simulink model "model"  (R2018a)
settings: Solver=VariableStepAuto  StartTime=0.0  StopTime=120  FixedStep=0.01  MaxStep=.001  RelTol=1e-3
libraries: instrumentlib x16, simulink x3
settings Model: Creator=U500304  LastModifiedBy=U500304
settings SolverCC: ZeroCrossAlgorithm=Adaptive
settings DebuggingCC: MaxConsecutiveZCsMsg=warning

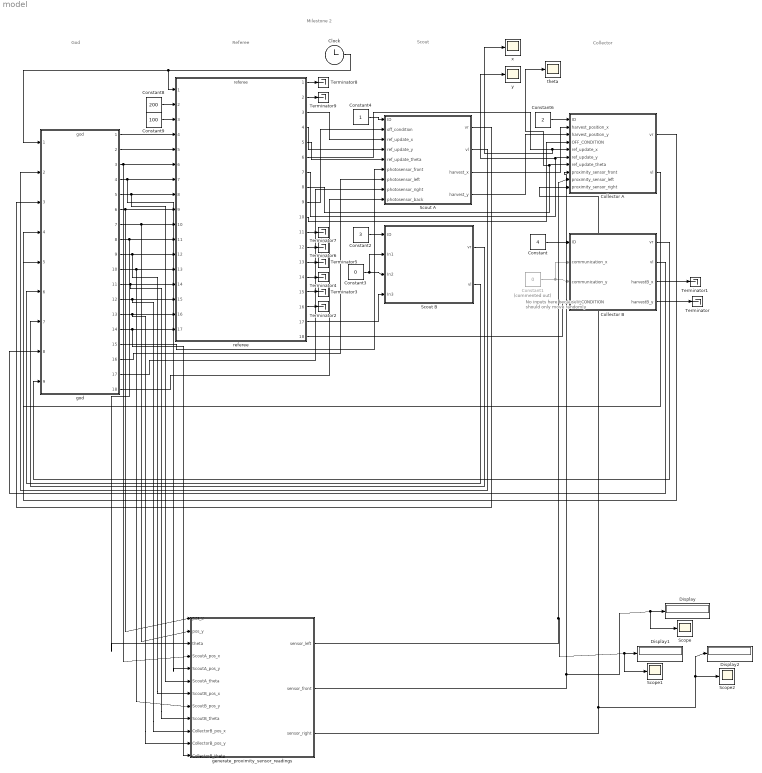
== system model ==
  note: No inputs here because
      | it should only move
      | randomly
  note: Milestone 2
  note: God
  note: Referee
  note: Scout
  note: Collector
  Clock : Clock
  Collector A : Subsystem
  Collector B : Subsystem
  Constant : Constant  Value=4
  Constant1 : Constant  Commented=on  Value=0
  Constant2 : Constant  Value=3
  Constant3 : Constant  Value=0
  Constant4 : Constant
  Constant6 : Constant  Value=2
  Constant8 : Constant  Value=200
  Constant9 : Constant  Value=100
  Display : Display
  Display1 : Display
  Display2 : Display
  Scope : Scope
  Scope1 : Scope
  Scope2 : Scope
  Scout A : Subsystem
  Scout B : Subsystem
  Terminator{,1..9} (10 alike) : Terminator
  generate_proximity_sensor_readings : Subsystem
  god : ModelReference  ModelNameDialog=god  SimulationMode=Normal  ModelReferenceVersion=1.469
  referee : ModelReference  ModelNameDialog=referee  SimulationMode=Normal  ModelReferenceVersion=1.290
  theta : Scope
  x : Scope
  y : Scope
  wires:
  Clock/1 -> god/1, referee/1
  Constant/1 -> Collector B/1(ID)
  Constant1/1 -> Collector B/2(communication_x), Collector B/3(communication_y)
  Constant2/1 -> Scout B/1(ID)
  Constant3/1 -> Scout B/2(In1), Scout B/3(In2)
  Constant4/1 -> Scout A/1(ID)
  Constant6/1 -> Collector A/1(ID)
  Constant8/1 -> referee/2
  Constant9/1 -> referee/3
  god/1 -> referee/4
  god/2 -> referee/5
  god/3 -> generate_proximity_sensor_readings/4(ScoutA_pos_x), referee/6
  god/5 -> generate_proximity_sensor_readings/6(ScoutA_theta), referee/8
  god/6 -> generate_proximity_sensor_readings/1(pos_x), referee/9
  god/7 -> generate_proximity_sensor_readings/2(pos_y), referee/10
  god/8 -> generate_proximity_sensor_readings/3(theta), referee/11
  god/9 -> generate_proximity_sensor_readings/7(ScoutB_pos_x), referee/12
  god/10 -> generate_proximity_sensor_readings/8(ScoutB_pos_y), referee/13
  god/11 -> generate_proximity_sensor_readings/9(ScoutB_theta), referee/14
  god/12 -> generate_proximity_sensor_readings/10(CollectorB_pos_x), referee/15
  god/14 -> generate_proximity_sensor_readings/12(CollectorB_theta), referee/17
  Scout B/2(vl) -> god/6
  Scout B/1(vr) -> god/7
  Collector A/2(vl) -> god/4
  Collector A/1(vr) -> god/5
  Collector B/1(vr) -> god/9
  Collector B/2(vl) -> god/8
  god/13 -> generate_proximity_sensor_readings/11(CollectorB_pos_y), referee/16
  god/4 -> generate_proximity_sensor_readings/5(ScoutA_pos_y), referee/7
  Scout A/1(vr) -> god/3
  Scout A/2(vl) -> god/2
  god/18 -> Scout A/9(photosensor_back)
  god/17 -> Scout A/8(photosensor_right)
  god/16 -> Scout A/7(photosensor_left)
  god/15 -> Scout A/6(photosensor_front)
  Scout A/3(harvest_x) -> Collector A/2(harvest_position_x)
  Scout A/4(harvest_y) -> Collector A/3(harvest_position_y)
  referee/3 -> Scout A/3(ref_update_x)
  referee/4 -> Scout A/4(ref_update_y)
  referee/5 -> Scout A/5(ref_update_theta)
  referee/6 -> x/1, Collector A/5(ref_update_x)
  referee/7 -> y/1, Collector A/6(ref_update_y)
  referee/8 -> theta/1, Collector A/7(ref_update_theta)
  referee/9 -> Scout A/2(off_condition)
  referee/10 -> Collector A/4(OFF_CONDITION)
  referee/18 -> Collector B/4(OFF_CONDITION)
  referee/17 -> Scout B/4(In3)
  generate_proximity_sensor_readings/1(sensor_left) -> Scope1/1, Display1/1, Collector A/9(proximity_sensor_left)
  generate_proximity_sensor_readings/2(sensor_front) -> Scope/1, Display/1, Collector A/8(proximity_sensor_front)
  generate_proximity_sensor_readings/3("sensor_right ") -> Scope2/1, Display2/1, Collector A/10(proximity_sensor_right)
  Collector B/4(harvestB_y) -> Terminator/1
  Collector B/3(harvestB_x) -> Terminator1/1
  referee/16 -> Terminator2/1
  referee/15 -> Terminator3/1
  referee/14 -> Terminator4/1
  referee/13 -> Terminator5/1
  referee/12 -> Terminator6/1
  referee/11 -> Terminator7/1
  referee/2 -> Terminator9/1
  referee/1 -> Terminator8/1

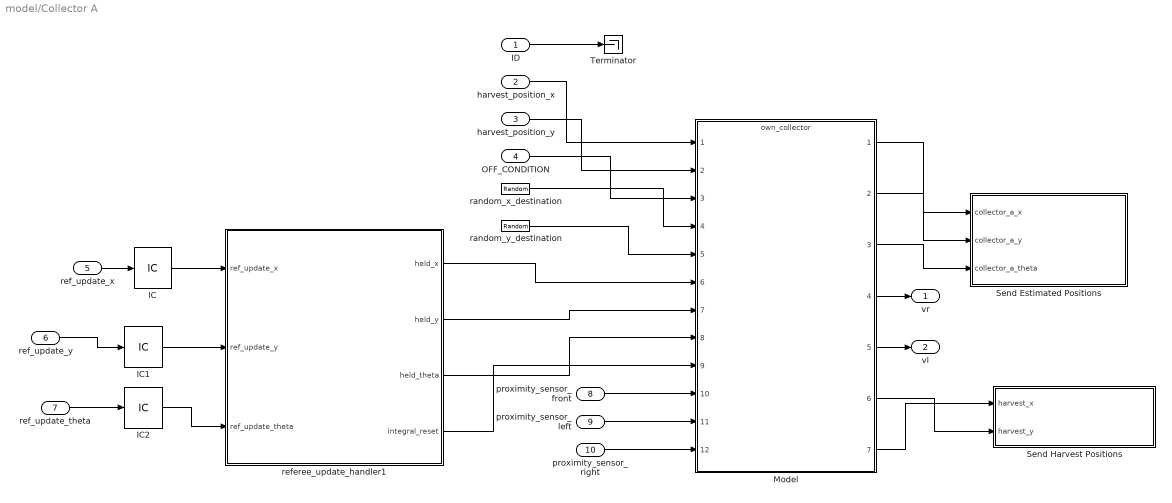
== system model/Collector A ==
  ID : Inport
  harvest_position_x : Inport  Port=2
  harvest_position_y : Inport  Port=3
  OFF_CONDITION : Inport  Port=4  OutDataTypeStr=boolean
  ref_update_x : Inport  Port=5
  ref_update_y : Inport  Port=6
  ref_update_theta : Inport  Port=7
  proximity_sensor_front : Inport  Port=8
  proximity_sensor_left : Inport  Port=9
  proximity_sensor_right : Inport  Port=10
  IC : InitialCondition  Value=0
  IC1 : InitialCondition  Value=49
  IC2 : InitialCondition  Value=0
  Model : ModelReference  ModelNameDialog=own_collector.slx  SimulationMode=Normal  ModelReferenceVersion=1.434
  Send Estimated Positions : Subsystem
  Send Harvest Positions : Subsystem
  Terminator : Terminator
  random_x_destination : UniformRandomNumber  Minimum=-3  Maximum=3  Seed=13  SampleTime=1
  random_y_destination : UniformRandomNumber  Minimum=-3  Maximum=3  Seed=15  SampleTime=1
  referee_update_handler1 : Subsystem
  vr : Outport
  vl : Outport  Port=2
  wires:
  ID/1 -> Terminator/1
  harvest_position_x/1 -> Model/1
  harvest_position_y/1 -> Model/2
  OFF_CONDITION/1 -> Model/3
  random_x_destination/1 -> Model/4
  random_y_destination/1 -> Model/5
  Model/4 -> vr/1
  Model/5 -> vl/1
  Model/1 -> Send Estimated Positions/1(collector_a_x)
  Model/2 -> Send Estimated Positions/2(collector_a_y)
  Model/3 -> Send Estimated Positions/3(collector_a_theta)
  Model/6 -> Send Harvest Positions/2(harvest_y)
  Model/7 -> Send Harvest Positions/1(harvest_x)
  ref_update_x/1 -> IC/1
  ref_update_y/1 -> IC1/1
  ref_update_theta/1 -> IC2/1
  referee_update_handler1/1(held_x) -> Model/6
  referee_update_handler1/2(held_y) -> Model/7
  referee_update_handler1/3(held_theta) -> Model/8
  referee_update_handler1/4(integral_reset) -> Model/9
  IC/1 -> referee_update_handler1/1(ref_update_x)
  IC1/1 -> referee_update_handler1/2(ref_update_y)
  IC2/1 -> referee_update_handler1/3(ref_update_theta)
  proximity_sensor_front/1 -> Model/10
  proximity_sensor_left/1 -> Model/11
  proximity_sensor_right/1 -> Model/12

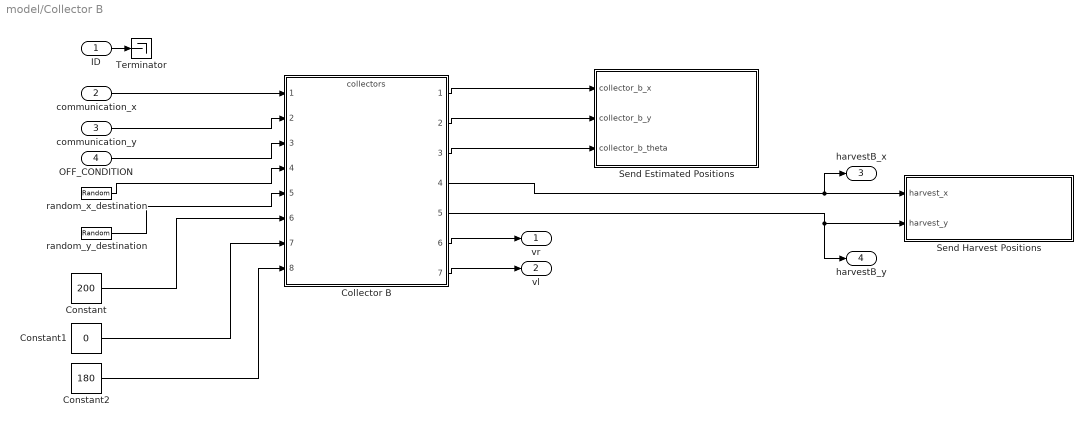
== system model/Collector B ==
  ID : Inport
  communication_x : Inport  Port=2
  communication_y : Inport  Port=3
  OFF_CONDITION : Inport  Port=4  OutDataTypeStr=boolean
  Collector B : ModelReference  ModelNameDialog=collectors  SimulationMode=Normal  ModelReferenceVersion=1.299
  Constant : Constant  Value=200
  Constant1 : Constant  Value=0
  Constant2 : Constant  Value=180
  Send Estimated Positions : Subsystem
  Send Harvest Positions : Subsystem
  Terminator : Terminator
  random_x_destination : UniformRandomNumber  Minimum=0  Maximum=199  Seed=18  SampleTime=1
  random_y_destination : UniformRandomNumber  Minimum=0  Maximum=99  Seed=19  SampleTime=1
  vr : Outport
  vl : Outport  Port=2
  harvestB_x : Outport  Port=3
  harvestB_y : Outport  Port=4
  wires:
  Collector B/2 -> Send Estimated Positions/2(collector_b_y)
  communication_x/1 -> Collector B/1
  Collector B/3 -> Send Estimated Positions/3(collector_b_theta)
  random_y_destination/1 -> Collector B/5
  random_x_destination/1 -> Collector B/4
  Collector B/1 -> Send Estimated Positions/1(collector_b_x)
  OFF_CONDITION/1 -> Collector B/3
  communication_y/1 -> Collector B/2
  ID/1 -> Terminator/1
  Collector B/6 -> vr/1
  Collector B/7 -> vl/1
  Collector B/4 -> harvestB_x/1, Send Harvest Positions/1(harvest_x)
  Collector B/5 -> harvestB_y/1, Send Harvest Positions/2(harvest_y)
  Constant/1 -> Collector B/6
  Constant1/1 -> Collector B/7
  Constant2/1 -> Collector B/8

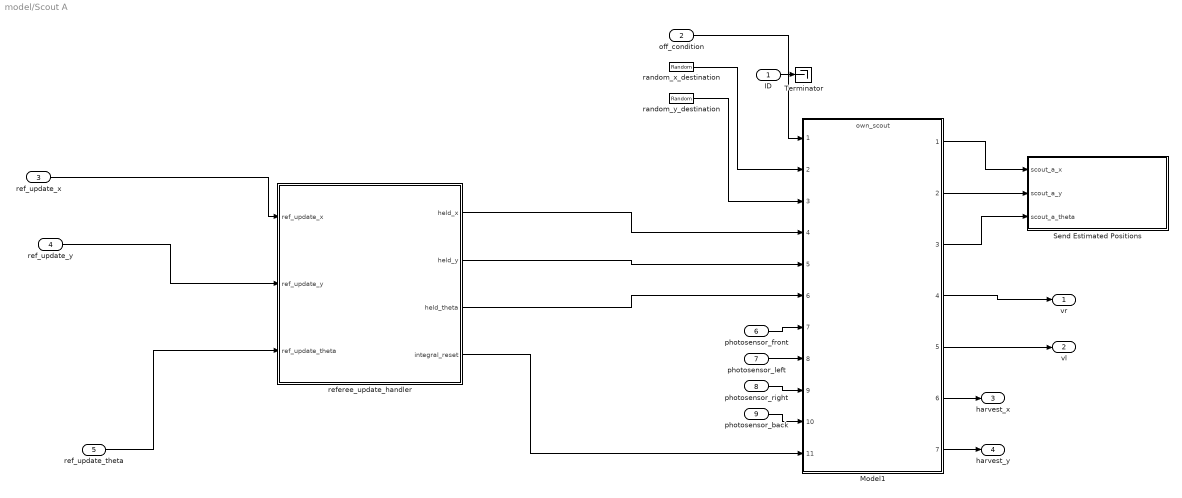
== system model/Scout A ==
  ID : Inport
  off_condition : Inport  Port=2  OutDataTypeStr=boolean
  ref_update_x : Inport  Port=3
  ref_update_y : Inport  Port=4
  ref_update_theta : Inport  Port=5
  photosensor_front : Inport  Port=6
  photosensor_left : Inport  Port=7
  photosensor_right : Inport  Port=8
  photosensor_back : Inport  Port=9
  Model1 : ModelReference  ModelNameDialog=own_scout.slx  SimulationMode=Normal  ModelReferenceVersion=1.295
  Send Estimated Positions : Subsystem
  Terminator : Terminator
  random_x_destination : UniformRandomNumber  Minimum=0  Maximum=199  Seed=11  SampleTime=1
  random_y_destination : UniformRandomNumber  Minimum=0  Maximum=99  Seed=12  SampleTime=1
  referee_update_handler : Subsystem
  vr : Outport
  vl : Outport  Port=2
  harvest_x : Outport  Port=3
  harvest_y : Outport  Port=4
  wires:
  off_condition/1 -> Model1/1
  random_x_destination/1 -> Model1/2
  random_y_destination/1 -> Model1/3
  ID/1 -> Terminator/1
  Model1/1 -> Send Estimated Positions/1(scout_a_x)
  Model1/2 -> Send Estimated Positions/2(scout_a_y)
  Model1/3 -> Send Estimated Positions/3(scout_a_theta)
  Model1/4 -> vr/1
  Model1/5 -> vl/1
  Model1/7 -> harvest_y/1
  Model1/6 -> harvest_x/1
  photosensor_back/1 -> Model1/10
  photosensor_right/1 -> Model1/9
  photosensor_left/1 -> Model1/8
  photosensor_front/1 -> Model1/7
  ref_update_x/1 -> referee_update_handler/1(ref_update_x)
  ref_update_y/1 -> referee_update_handler/2(ref_update_y)
  ref_update_theta/1 -> referee_update_handler/3(ref_update_theta)
  referee_update_handler/1(held_x) -> Model1/4
  referee_update_handler/2(held_y) -> Model1/5
  referee_update_handler/3(held_theta) -> Model1/6
  referee_update_handler/4(integral_reset) -> Model1/11

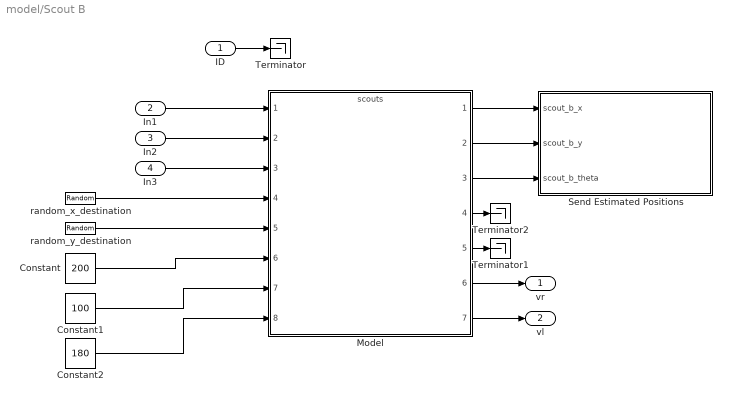
== system model/Scout B ==
  ID : Inport
  In1 : Inport  Port=2
  In2 : Inport  Port=3
  In3 : Inport  Port=4  OutDataTypeStr=boolean
  Constant : Constant  Value=200
  Constant1 : Constant  Value=100
  Constant2 : Constant  Value=180
  Model : ModelReference  ModelNameDialog=scouts.slx  SimulationMode=Normal  ModelReferenceVersion=1.251
  Send Estimated Positions : Subsystem
  Terminator : Terminator
  Terminator1 : Terminator
  Terminator2 : Terminator
  random_x_destination : UniformRandomNumber  Minimum=0  Maximum=199  Seed=16  SampleTime=1
  random_y_destination : UniformRandomNumber  Minimum=0  Maximum=99  Seed=17  SampleTime=1
  vr : Outport
  vl : Outport  Port=2
  wires:
  random_y_destination/1 -> Model/5
  random_x_destination/1 -> Model/4
  In3/1 -> Model/3
  Model/2 -> Send Estimated Positions/2(scout_b_y)
  Model/1 -> Send Estimated Positions/1(scout_b_x)
  In1/1 -> Model/1
  In2/1 -> Model/2
  Model/3 -> Send Estimated Positions/3(scout_b_theta)
  ID/1 -> Terminator/1
  Model/6 -> vr/1
  Model/7 -> vl/1
  Model/4 -> Terminator2/1
  Model/5 -> Terminator1/1
  Constant/1 -> Model/6
  Constant1/1 -> Model/7
  Constant2/1 -> Model/8

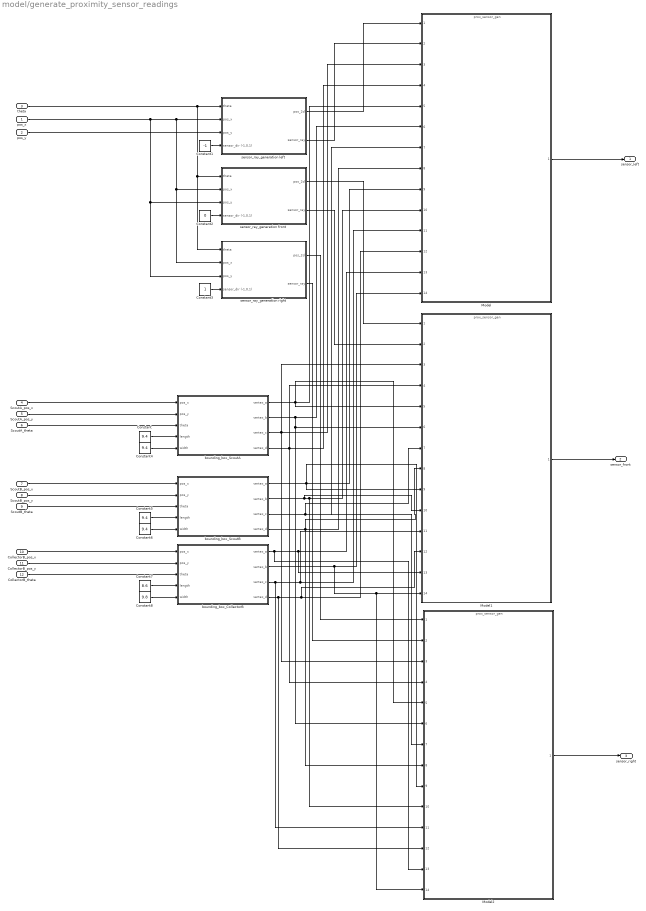
== system model/generate_proximity_sensor_readings ==
  pos_x : Inport
  pos_y : Inport  Port=2
  theta : Inport  Port=3
  ScoutA_pos_x : Inport  Port=4
  ScoutA_pos_y : Inport  Port=5
  ScoutA_theta : Inport  Port=6
  ScoutB_pos_x : Inport  Port=7
  ScoutB_pos_y : Inport  Port=8
  ScoutB_theta : Inport  Port=9
  CollectorB_pos_x : Inport  Port=10
  CollectorB_pos_y : Inport  Port=11
  CollectorB_theta : Inport  Port=12
  Constant{,4..6} (4 alike) : Constant  Value=9.4
  Constant1 : Constant  Value=-1
  Constant2 : Constant  Value=0
  Constant3 : Constant
  Constant7 : Constant  Value=8.6
  Constant8 : Constant  Value=9.8
  Model : ModelReference  ModelNameDialog=prox_sensor_gen  SimulationMode=Normal  ModelReferenceVersion=1.2
  Model1 : ModelReference  ModelNameDialog=prox_sensor_gen  SimulationMode=Normal  ModelReferenceVersion=1.2
  Model2 : ModelReference  ModelNameDialog=prox_sensor_gen  SimulationMode=Normal  ModelReferenceVersion=1.2
  bounding_box_CollectorB : Subsystem
  bounding_box_ScoutA : Subsystem
  bounding_box_ScoutB : Subsystem
  sensor_ray_generation front : Subsystem
  sensor_ray_generation left : Subsystem
  sensor_ray_generation right : Subsystem
  sensor_left : Outport
  sensor_front : Outport  Port=2
  "sensor_right " : Outport  Port=3
  wires:
  theta/1 -> sensor_ray_generation right/1("theta "), sensor_ray_generation front/1("theta "), sensor_ray_generation left/1("theta ")
  bounding_box_CollectorB/2(vertex_b) -> Model/14, Model2/14, Model1/14
  Constant2/1 -> sensor_ray_generation front/4("sensor_dir (-1,0,1) ")
  Model2/1 -> "sensor_right "/1
  bounding_box_ScoutB/4(vertex_d) -> Model2/8, Model1/8, Model/8
  Constant8/1 -> bounding_box_CollectorB/5(width)
  bounding_box_ScoutA/1(vertex_a) -> Model2/5, Model1/5, Model/5
  bounding_box_CollectorB/3(vertex_c) -> Model2/11, Model1/11, Model/11
  ScoutB_theta/1 -> bounding_box_ScoutB/3(theta)
  Constant5/1 -> bounding_box_ScoutB/4(length)
  ScoutA_pos_x/1 -> bounding_box_ScoutA/1(pos_x)
  bounding_box_ScoutA/3(vertex_c) -> Model2/3, Model1/3, Model/3
  Constant6/1 -> bounding_box_ScoutB/5(width)
  Constant1/1 -> sensor_ray_generation left/4("sensor_dir (-1,0,1) ")
  bounding_box_CollectorB/1(vertex_a) -> Model2/13, Model1/13, Model/13
  bounding_box_ScoutA/4(vertex_d) -> Model2/4, Model1/4, Model/4
  sensor_ray_generation front/1(pos_2d) -> Model1/1
  sensor_ray_generation left/2("sensor_ray ") -> Model/2
  bounding_box_CollectorB/4(vertex_d) -> Model2/12, Model1/12, Model/12
  ScoutB_pos_y/1 -> bounding_box_ScoutB/2(pos_y)
  Model/1 -> sensor_left/1
  pos_y/1 -> sensor_ray_generation left/3(pos_y)
  bounding_box_ScoutB/2(vertex_b) -> Model1/10, Model2/10, Model/10
  Model1/1 -> sensor_front/1
  bounding_box_ScoutB/1(vertex_a) -> Model2/9, Model1/9, Model/9
  bounding_box_ScoutA/2(vertex_b) -> Model/6, Model2/6, Model1/6
  bounding_box_ScoutB/3(vertex_c) -> Model2/7, Model1/7, Model/7
  sensor_ray_generation right/2("sensor_ray ") -> Model2/2
  ScoutA_pos_y/1 -> bounding_box_ScoutA/2(pos_y)
  CollectorB_theta/1 -> bounding_box_CollectorB/3(theta)
  pos_x/1 -> sensor_ray_generation right/3(pos_y), sensor_ray_generation front/3(pos_y), sensor_ray_generation right/2(pos_x), sensor_ray_generation front/2(pos_x), sensor_ray_generation left/2(pos_x)
  sensor_ray_generation right/1(pos_2d) -> Model2/1
  Constant4/1 -> bounding_box_ScoutA/5(width)
  CollectorB_pos_x/1 -> bounding_box_CollectorB/1(pos_x)
  Constant/1 -> bounding_box_ScoutA/4(length)
  CollectorB_pos_y/1 -> bounding_box_CollectorB/2(pos_y)
  Constant7/1 -> bounding_box_CollectorB/4(length)
  ScoutA_theta/1 -> bounding_box_ScoutA/3(theta)
  ScoutB_pos_x/1 -> bounding_box_ScoutB/1(pos_x)
  Constant3/1 -> sensor_ray_generation right/4("sensor_dir (-1,0,1) ")
  sensor_ray_generation left/1(pos_2d) -> Model/1
  sensor_ray_generation front/2("sensor_ray ") -> Model1/2

== system model/Collector A/Send Estimated Positions ==
  note: Collector
  collector_a_x : Inport
  collector_a_y : Inport  Port=2
  collector_a_theta : Inport  Port=3
  Rate Transition : RateTransition  OutPortSampleTime=0.05
  Rate Transition1 : RateTransition  OutPortSampleTime=0.05
  Rate Transition2 : RateTransition  OutPortSampleTime=0.05
  tcp_send_collector_a_theta : instrumentlib/TCP//IP Send  Host=localhost  Port=50006  EnableBlockingMode=off  Timeout=1  ByteOrder=LittleEndian  TransferDelay=on
      settings: SourceProductName=Instrument Control Toolbox
  tcp_send_collector_a_x : instrumentlib/TCP//IP Send  Host=localhost  Port=50004  EnableBlockingMode=off  Timeout=1  ByteOrder=LittleEndian  TransferDelay=on
      settings: SourceProductName=Instrument Control Toolbox
  tcp_send_collector_a_y : instrumentlib/TCP//IP Send  Host=localhost  Port=50005  EnableBlockingMode=off  Timeout=1  ByteOrder=LittleEndian  TransferDelay=on
      settings: SourceProductName=Instrument Control Toolbox
  wires:
  collector_a_x/1 -> Rate Transition/1
  collector_a_y/1 -> Rate Transition1/1
  collector_a_theta/1 -> Rate Transition2/1
  Rate Transition/1 -> tcp_send_collector_a_x/1
  Rate Transition1/1 -> tcp_send_collector_a_y/1
  Rate Transition2/1 -> tcp_send_collector_a_theta/1

== system model/Collector A/Send Harvest Positions ==
  note: Collector
  harvest_x : Inport
  harvest_y : Inport  Port=2
  Rate Transition3 : RateTransition  OutPortSampleTime=0.5
  Rate Transition4 : RateTransition  OutPortSampleTime=0.5
  tcp_send_harvest_a_x : instrumentlib/TCP//IP Send  Host=localhost  Port=50025  EnableBlockingMode=off  Timeout=1  ByteOrder=LittleEndian  TransferDelay=on
      settings: SourceProductName=Instrument Control Toolbox
  tcp_send_harvest_a_y : instrumentlib/TCP//IP Send  Host=localhost  Port=50026  EnableBlockingMode=off  Timeout=1  ByteOrder=LittleEndian  TransferDelay=on
      settings: SourceProductName=Instrument Control Toolbox
  wires:
  Rate Transition3/1 -> tcp_send_harvest_a_x/1
  harvest_x/1 -> Rate Transition3/1
  harvest_y/1 -> Rate Transition4/1
  Rate Transition4/1 -> tcp_send_harvest_a_y/1

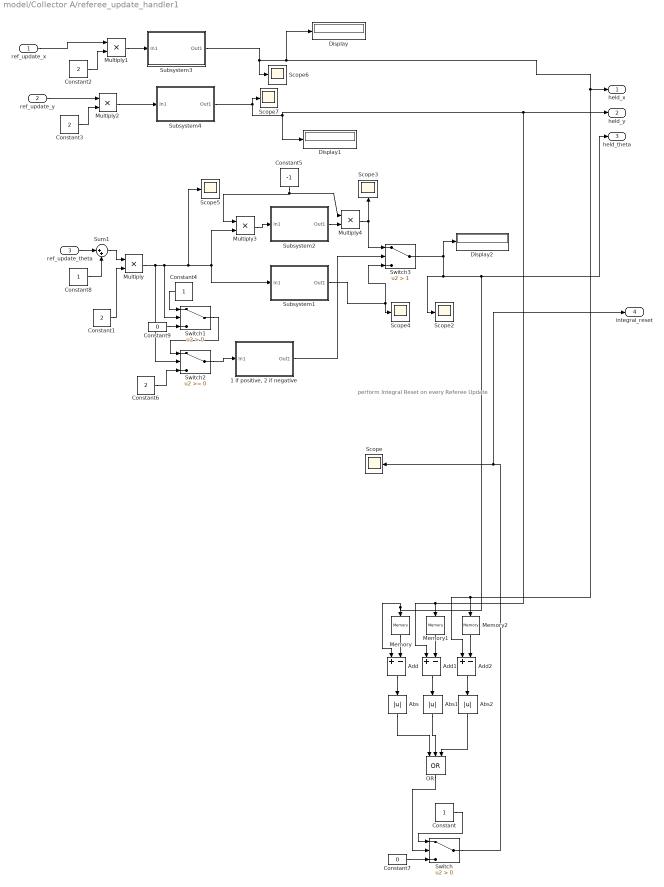
== system model/Collector A/referee_update_handler1 ==
  note: perform
      | Integral
      | Reset on
      | every
      | Referee
      | Update
  ref_update_x : Inport
  ref_update_y : Inport  Port=2
  ref_update_theta : Inport  Port=3
  "1 if positive, 2 if negative" : Subsystem
  Abs : Abs
  Abs1 : Abs
  Abs2 : Abs
  Add : Sum  Inputs=+-
  Add1 : Sum  Inputs=+-
  Add2 : Sum  Inputs=+-
  Constant : Constant
  Constant{1..3,6} (4 alike) : Constant  Value=2
  Constant4 : Constant
  Constant5 : Constant  Value=-1
  Constant7 : Constant  Value=0
  Constant8 : Constant
  Constant9 : Constant  Value=0
  Display : Display
  Display1 : Display
  Display2 : Display
  Memory : Memory
  Memory1 : Memory
  Memory2 : Memory
  Multiply{,1..4} (5 alike) : Product
  OR : Logic  Operator=OR  Inputs=3  IconShape=distinctive  AllPortsSameDT=off  OutDataTypeStr=boolean
  Scope{,2..7} (7 alike) : Scope
  Subsystem1 : Subsystem
  Subsystem2 : Subsystem
  Subsystem3 : Subsystem
  Subsystem4 : Subsystem
  Sum1 : Sum  Inputs=|++
  Switch : Switch  Criteria=u2 > Threshold
  Switch1 : Switch  Criteria=u2 > Threshold
  Switch2 : Switch
  Switch3 : Switch  Criteria=u2 > Threshold  Threshold=1
  held_x : Outport
  held_y : Outport  Port=2
  held_theta : Outport  Port=3
  integral_reset : Outport  Port=4
  wires:
  Multiply1/1 -> Subsystem3/1(In1)
  Add/1 -> Abs/1
  Subsystem3/1(Out1) -> Scope6/1, held_x/1, Add2/1, Memory2/1, Display/1
  Constant1/1 -> Multiply/2
  Subsystem2/1(Out1) -> Multiply4/2
  Multiply3/1 -> Subsystem2/1(In1)
  Multiply/1 -> Switch2/2, Switch1/2, Multiply3/2, Subsystem1/1(In1), Scope5/1
  Subsystem4/1(Out1) -> held_y/1, Add1/1, Memory1/1, Display1/1, Scope7/1
  Constant6/1 -> Switch2/3
  Add2/1 -> Abs2/1
  Memory2/1 -> Add2/2
  Constant3/1 -> Multiply2/2
  Switch3/1 -> Scope2/1, held_theta/1, Add/1, Memory/1, Display2/1
  "1 if positive, 2 if negative"/1(Out1) -> Switch3/2
  Constant2/1 -> Multiply1/2
  Constant5/1 -> Multiply4/1, Multiply3/1
  Switch1/1 -> Switch2/1
  Multiply4/1 -> Scope3/1, Switch3/1
  Sum1/1 -> Multiply/1
  Switch/1 -> integral_reset/1, Scope/1
  Abs2/1 -> OR/3
  Multiply2/1 -> Subsystem4/1(In1)
  Constant/1 -> Switch/1
  Subsystem1/1(Out1) -> Switch3/3, Scope4/1
  Memory/1 -> Add/2
  ref_update_x/1 -> Multiply1/1
  Abs/1 -> OR/1
  ref_update_theta/1 -> Sum1/1
  ref_update_y/1 -> Multiply2/1
  OR/1 -> Switch/2
  Abs1/1 -> OR/2
  Constant8/1 -> Sum1/2
  Add1/1 -> Abs1/1
  Memory1/1 -> Add1/2
  Constant4/1 -> Switch1/1
  Switch2/1 -> "1 if positive, 2 if negative"/1(In1)
  Constant7/1 -> Switch/3
  Constant9/1 -> Switch1/3

== system model/Collector B/Send Estimated Positions ==
  note: Collector
  collector_b_x : Inport
  collector_b_y : Inport  Port=2
  collector_b_theta : Inport  Port=3
  Rate Transition10 : RateTransition  OutPortSampleTime=0.1
  Rate Transition11 : RateTransition  OutPortSampleTime=0.1
  Rate Transition9 : RateTransition  OutPortSampleTime=0.1
  tcp_send_collector_b_theta : instrumentlib/TCP//IP Send  Host=localhost  Port=50012  EnableBlockingMode=off  Timeout=1  ByteOrder=LittleEndian  TransferDelay=on
      settings: SourceProductName=Instrument Control Toolbox
  tcp_send_collector_b_x : instrumentlib/TCP//IP Send  Host=localhost  Port=50010  EnableBlockingMode=off  Timeout=1  ByteOrder=LittleEndian  TransferDelay=on
      settings: SourceProductName=Instrument Control Toolbox
  tcp_send_collector_b_y : instrumentlib/TCP//IP Send  Host=localhost  Port=50011  EnableBlockingMode=off  Timeout=1  ByteOrder=LittleEndian  TransferDelay=on
      settings: SourceProductName=Instrument Control Toolbox
  wires:
  collector_b_x/1 -> Rate Transition9/1
  collector_b_y/1 -> Rate Transition10/1
  collector_b_theta/1 -> Rate Transition11/1
  Rate Transition9/1 -> tcp_send_collector_b_x/1
  Rate Transition10/1 -> tcp_send_collector_b_y/1
  Rate Transition11/1 -> tcp_send_collector_b_theta/1

== system model/Collector B/Send Harvest Positions ==
  note: Collector
  harvest_x : Inport
  harvest_y : Inport  Port=2
  Rate Transition3 : RateTransition  OutPortSampleTime=0.5
  Rate Transition4 : RateTransition  OutPortSampleTime=0.5
  tcp_send_collector_b_theta2 : instrumentlib/TCP//IP Send  Host=localhost  Port=50028  EnableBlockingMode=off  Timeout=1  ByteOrder=LittleEndian  TransferDelay=on
      settings: SourceProductName=Instrument Control Toolbox
  tcp_send_harvest_b_x : instrumentlib/TCP//IP Send  Host=localhost  Port=50027  EnableBlockingMode=off  Timeout=1  ByteOrder=LittleEndian  TransferDelay=on
      settings: SourceProductName=Instrument Control Toolbox
  wires:
  Rate Transition3/1 -> tcp_send_harvest_b_x/1
  harvest_x/1 -> Rate Transition3/1
  harvest_y/1 -> Rate Transition4/1
  Rate Transition4/1 -> tcp_send_collector_b_theta2/1

== system model/Scout A/Send Estimated Positions ==
  note: Scout
  scout_a_x : Inport
  scout_a_y : Inport  Port=2
  scout_a_theta : Inport  Port=3
  Rate Transition5 : RateTransition  OutPortSampleTime=0.05
  Rate Transition6 : RateTransition  OutPortSampleTime=0.05
  Rate Transition7 : RateTransition  OutPortSampleTime=0.05
  tcp_send_scout_a_theta : instrumentlib/TCP//IP Send  Host=localhost  Port=50003  EnableBlockingMode=off  Timeout=1  ByteOrder=LittleEndian  TransferDelay=on
      settings: SourceProductName=Instrument Control Toolbox
  tcp_send_scout_a_x : instrumentlib/TCP//IP Send  Host=localhost  Port=50001  EnableBlockingMode=off  Timeout=1  ByteOrder=LittleEndian  TransferDelay=on
      settings: SourceProductName=Instrument Control Toolbox
  tcp_send_scout_a_y : instrumentlib/TCP//IP Send  Host=localhost  Port=50002  EnableBlockingMode=off  Timeout=1  ByteOrder=LittleEndian  TransferDelay=on
      settings: SourceProductName=Instrument Control Toolbox
  wires:
  scout_a_x/1 -> Rate Transition5/1
  scout_a_y/1 -> Rate Transition6/1
  scout_a_theta/1 -> Rate Transition7/1
  Rate Transition5/1 -> tcp_send_scout_a_x/1
  Rate Transition6/1 -> tcp_send_scout_a_y/1
  Rate Transition7/1 -> tcp_send_scout_a_theta/1

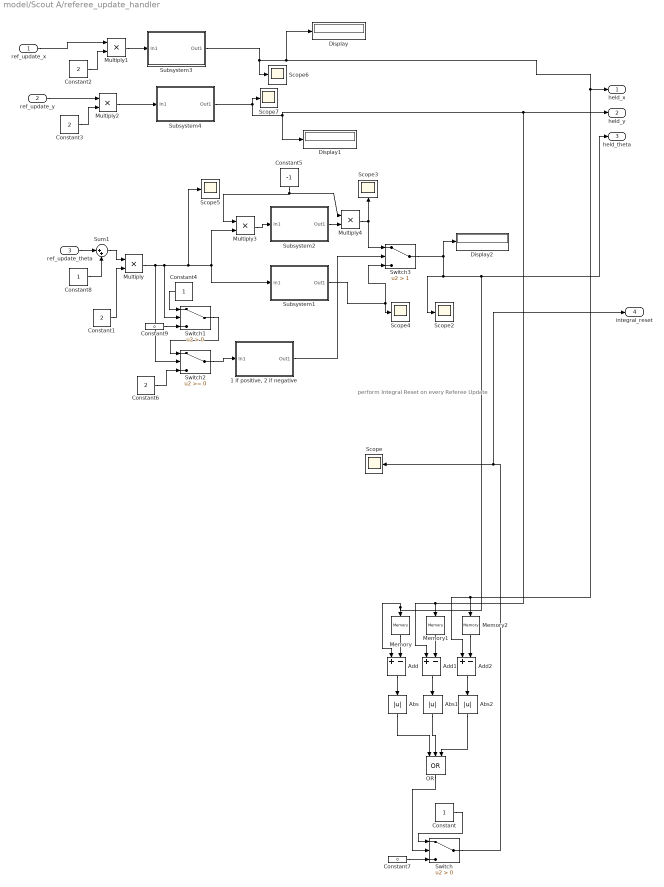
== system model/Scout A/referee_update_handler ==
  note: perform
      | Integral
      | Reset on
      | every
      | Referee
      | Update
  ref_update_x : Inport
  ref_update_y : Inport  Port=2
  ref_update_theta : Inport  Port=3
  "1 if positive, 2 if negative" : Subsystem
  Abs : Abs
  Abs1 : Abs
  Abs2 : Abs
  Add : Sum  Inputs=+-
  Add1 : Sum  Inputs=+-
  Add2 : Sum  Inputs=+-
  Constant : Constant
  Constant{1..3,6} (4 alike) : Constant  Value=2
  Constant4 : Constant
  Constant5 : Constant  Value=-1
  Constant7 : Constant  Value=0
  Constant8 : Constant
  Constant9 : Constant  Value=0
  Display : Display
  Display1 : Display
  Display2 : Display
  Memory : Memory
  Memory1 : Memory
  Memory2 : Memory
  Multiply{,1..4} (5 alike) : Product
  OR : Logic  Operator=OR  Inputs=3  IconShape=distinctive  AllPortsSameDT=off  OutDataTypeStr=boolean
  Scope{,2..7} (7 alike) : Scope
  Subsystem1 : Subsystem
  Subsystem2 : Subsystem
  Subsystem3 : Subsystem
  Subsystem4 : Subsystem
  Sum1 : Sum  Inputs=|++
  Switch : Switch  Criteria=u2 > Threshold
  Switch1 : Switch  Criteria=u2 > Threshold
  Switch2 : Switch
  Switch3 : Switch  Criteria=u2 > Threshold  Threshold=1
  held_x : Outport
  held_y : Outport  Port=2
  held_theta : Outport  Port=3
  integral_reset : Outport  Port=4
  wires:
  Multiply1/1 -> Subsystem3/1(In1)
  Add/1 -> Abs/1
  Subsystem3/1(Out1) -> Scope6/1, held_x/1, Add2/1, Memory2/1, Display/1
  Constant1/1 -> Multiply/2
  Subsystem2/1(Out1) -> Multiply4/2
  Multiply3/1 -> Subsystem2/1(In1)
  Multiply/1 -> Switch2/2, Switch1/2, Multiply3/2, Subsystem1/1(In1), Scope5/1
  Subsystem4/1(Out1) -> held_y/1, Add1/1, Memory1/1, Display1/1, Scope7/1
  Constant6/1 -> Switch2/3
  Add2/1 -> Abs2/1
  Memory2/1 -> Add2/2
  Constant3/1 -> Multiply2/2
  Switch3/1 -> Scope2/1, held_theta/1, Add/1, Memory/1, Display2/1
  "1 if positive, 2 if negative"/1(Out1) -> Switch3/2
  Constant2/1 -> Multiply1/2
  Constant5/1 -> Multiply4/1, Multiply3/1
  Switch1/1 -> Switch2/1
  Multiply4/1 -> Scope3/1, Switch3/1
  Sum1/1 -> Multiply/1
  Switch/1 -> integral_reset/1, Scope/1
  Abs2/1 -> OR/3
  Multiply2/1 -> Subsystem4/1(In1)
  Constant/1 -> Switch/1
  Subsystem1/1(Out1) -> Switch3/3, Scope4/1
  Memory/1 -> Add/2
  ref_update_x/1 -> Multiply1/1
  Abs/1 -> OR/1
  ref_update_theta/1 -> Sum1/1
  ref_update_y/1 -> Multiply2/1
  OR/1 -> Switch/2
  Abs1/1 -> OR/2
  Constant8/1 -> Sum1/2
  Add1/1 -> Abs1/1
  Memory1/1 -> Add1/2
  Constant4/1 -> Switch1/1
  Switch2/1 -> "1 if positive, 2 if negative"/1(In1)
  Constant7/1 -> Switch/3
  Constant9/1 -> Switch1/3

== system model/Scout B/Send Estimated Positions ==
  note: Scout
  scout_b_x : Inport
  scout_b_y : Inport  Port=2
  scout_b_theta : Inport  Port=3
  Rate Transition3 : RateTransition  OutPortSampleTime=0.1
  Rate Transition4 : RateTransition  OutPortSampleTime=0.1
  Rate Transition8 : RateTransition  OutPortSampleTime=0.1
  tcp_send_scout_b_theta : instrumentlib/TCP//IP Send  Host=localhost  Port=50009  EnableBlockingMode=off  Timeout=1  ByteOrder=LittleEndian  TransferDelay=on
      settings: SourceProductName=Instrument Control Toolbox
  tcp_send_scout_b_x : instrumentlib/TCP//IP Send  Host=localhost  Port=50007  EnableBlockingMode=off  Timeout=1  ByteOrder=LittleEndian  TransferDelay=on
      settings: SourceProductName=Instrument Control Toolbox
  tcp_send_scout_b_y : instrumentlib/TCP//IP Send  Host=localhost  Port=50008  EnableBlockingMode=off  Timeout=1  ByteOrder=LittleEndian  TransferDelay=on
      settings: SourceProductName=Instrument Control Toolbox
  wires:
  scout_b_theta/1 -> Rate Transition8/1
  scout_b_y/1 -> Rate Transition4/1
  scout_b_x/1 -> Rate Transition3/1
  Rate Transition3/1 -> tcp_send_scout_b_x/1
  Rate Transition4/1 -> tcp_send_scout_b_y/1
  Rate Transition8/1 -> tcp_send_scout_b_theta/1

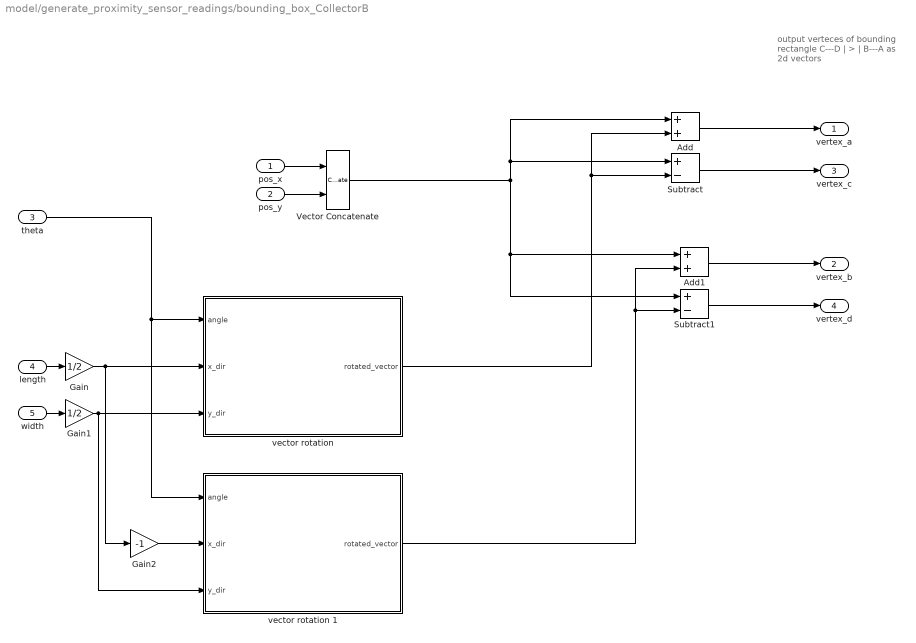
== system model/generate_proximity_sensor_readings/bounding_box_CollectorB ==
  note: output verteces of
      | bounding rectangle
      | C---D
      | |  >  |
      | B---A  as 2d vectors
  pos_x : Inport
  pos_y : Inport  Port=2
  theta : Inport  Port=3
  length : Inport  Port=4
  width : Inport  Port=5
  Add : Sum
  Add1 : Sum
  Gain : Gain  Gain=1/2
  Gain1 : Gain  Gain=1/2
  Gain2 : Gain  Gain=-1
  Subtract : Sum  Inputs=+-
  Subtract1 : Sum  Inputs=+-
  Vector Concatenate : Concatenate
  "vector rotation " : Subsystem
  vector rotation 1 : Subsystem
  vertex_a : Outport
  vertex_b : Outport  Port=2
  vertex_c : Outport  Port=3
  vertex_d : Outport  Port=4
  wires:
  Subtract1/1 -> vertex_d/1
  Add1/1 -> vertex_b/1
  Subtract/1 -> vertex_c/1
  Add/1 -> vertex_a/1
  vector rotation 1/1("rotated_vector ") -> Add1/2, Subtract1/2
  "vector rotation "/1("rotated_vector ") -> Add/2, Subtract/2
  Vector Concatenate/1 -> Add/1, Subtract/1, Add1/1, Subtract1/1
  Gain1/1 -> "vector rotation "/3(y_dir), vector rotation 1/3(y_dir)
  Gain2/1 -> vector rotation 1/2(x_dir)
  Gain/1 -> "vector rotation "/2(x_dir), Gain2/1
  theta/1 -> "vector rotation "/1(angle), vector rotation 1/1(angle)
  pos_y/1 -> Vector Concatenate/2
  pos_x/1 -> Vector Concatenate/1
  length/1 -> Gain/1
  width/1 -> Gain1/1

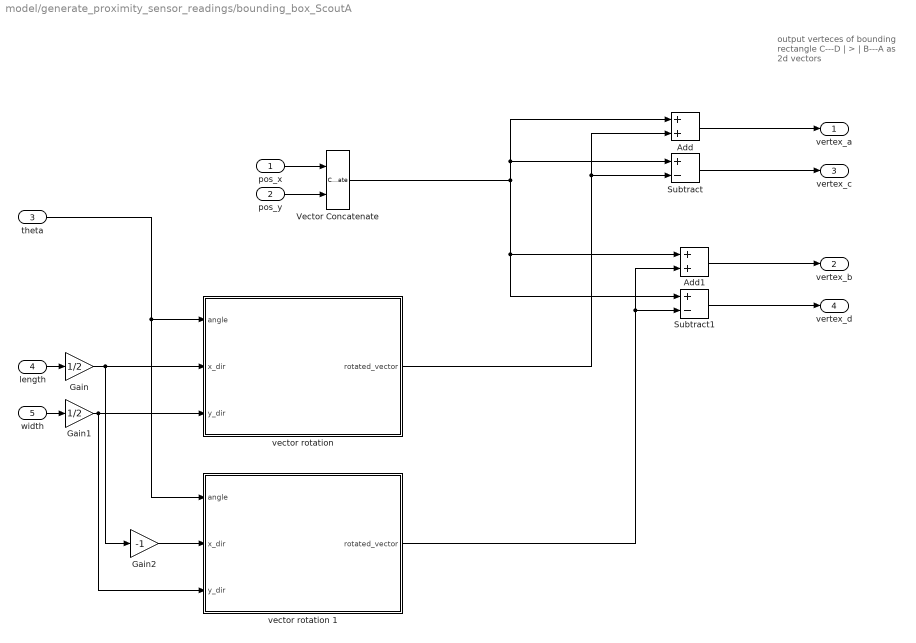
== system model/generate_proximity_sensor_readings/bounding_box_ScoutA ==
  note: output verteces of
      | bounding rectangle
      | C---D
      | |  >  |
      | B---A  as 2d vectors
  pos_x : Inport
  pos_y : Inport  Port=2
  theta : Inport  Port=3
  length : Inport  Port=4
  width : Inport  Port=5
  Add : Sum
  Add1 : Sum
  Gain : Gain  Gain=1/2
  Gain1 : Gain  Gain=1/2
  Gain2 : Gain  Gain=-1
  Subtract : Sum  Inputs=+-
  Subtract1 : Sum  Inputs=+-
  Vector Concatenate : Concatenate
  "vector rotation " : Subsystem
  vector rotation 1 : Subsystem
  vertex_a : Outport
  vertex_b : Outport  Port=2
  vertex_c : Outport  Port=3
  vertex_d : Outport  Port=4
  wires:
  Subtract1/1 -> vertex_d/1
  Add1/1 -> vertex_b/1
  Subtract/1 -> vertex_c/1
  Add/1 -> vertex_a/1
  vector rotation 1/1("rotated_vector ") -> Add1/2, Subtract1/2
  "vector rotation "/1("rotated_vector ") -> Add/2, Subtract/2
  Vector Concatenate/1 -> Add/1, Subtract/1, Add1/1, Subtract1/1
  Gain1/1 -> "vector rotation "/3(y_dir), vector rotation 1/3(y_dir)
  Gain2/1 -> vector rotation 1/2(x_dir)
  Gain/1 -> "vector rotation "/2(x_dir), Gain2/1
  theta/1 -> "vector rotation "/1(angle), vector rotation 1/1(angle)
  pos_y/1 -> Vector Concatenate/2
  pos_x/1 -> Vector Concatenate/1
  length/1 -> Gain/1
  width/1 -> Gain1/1

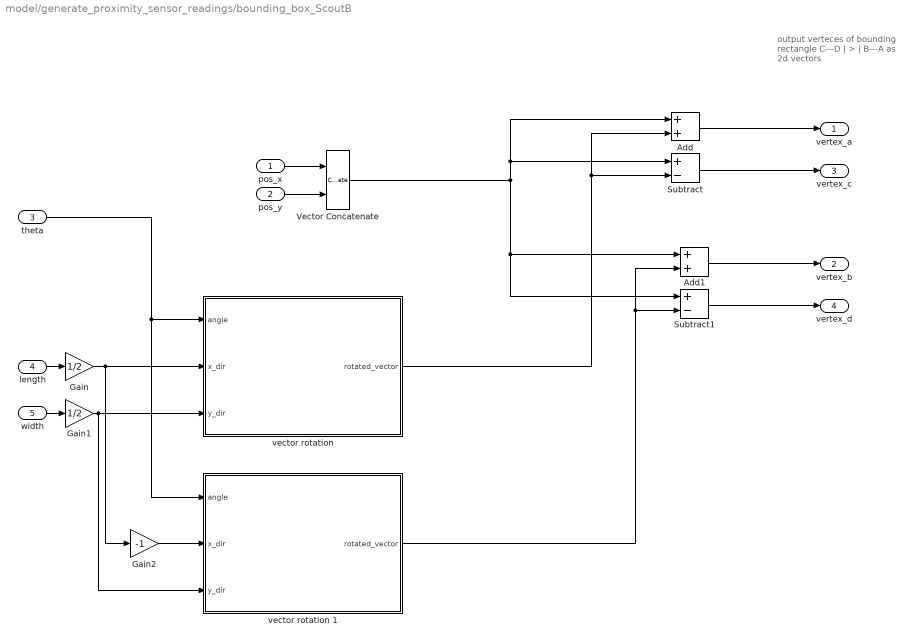
== system model/generate_proximity_sensor_readings/bounding_box_ScoutB ==
  note: output verteces of
      | bounding rectangle
      | C---D
      | |  >  |
      | B---A  as 2d vectors
  pos_x : Inport
  pos_y : Inport  Port=2
  theta : Inport  Port=3
  length : Inport  Port=4
  width : Inport  Port=5
  Add : Sum
  Add1 : Sum
  Gain : Gain  Gain=1/2
  Gain1 : Gain  Gain=1/2
  Gain2 : Gain  Gain=-1
  Subtract : Sum  Inputs=+-
  Subtract1 : Sum  Inputs=+-
  Vector Concatenate : Concatenate
  "vector rotation " : Subsystem
  vector rotation 1 : Subsystem
  vertex_a : Outport
  vertex_b : Outport  Port=2
  vertex_c : Outport  Port=3
  vertex_d : Outport  Port=4
  wires:
  width/1 -> Gain1/1
  length/1 -> Gain/1
  pos_x/1 -> Vector Concatenate/1
  pos_y/1 -> Vector Concatenate/2
  theta/1 -> vector rotation 1/1(angle), "vector rotation "/1(angle)
  Gain/1 -> Gain2/1, "vector rotation "/2(x_dir)
  Gain2/1 -> vector rotation 1/2(x_dir)
  Gain1/1 -> vector rotation 1/3(y_dir), "vector rotation "/3(y_dir)
  Vector Concatenate/1 -> Subtract1/1, Add1/1, Subtract/1, Add/1
  "vector rotation "/1("rotated_vector ") -> Subtract/2, Add/2
  vector rotation 1/1("rotated_vector ") -> Subtract1/2, Add1/2
  Add/1 -> vertex_a/1
  Subtract/1 -> vertex_c/1
  Add1/1 -> vertex_b/1
  Subtract1/1 -> vertex_d/1

== system model/generate_proximity_sensor_readings/sensor_ray_generation front ==
  "theta " : Inport
  pos_x : Inport  Port=2
  pos_y : Inport  Port=3
  "sensor_dir (-1,0,1) " : Inport  Port=4
  Compare To Zero : simulink/Logic and Bit Operations/Compare To Zero  relop===  OutDataTypeStr=boolean
  Constant : Constant  Value=1.0
  Constant1 : Constant  Value=0
  Switch : Switch  Threshold=1
  Vector Concatenate : Concatenate
  "vector rotation " : Subsystem
  pos_2d : Outport
  "sensor_ray " : Outport  Port=2
  wires:
  "vector rotation "/1("rotated_vector ") -> "sensor_ray "/1
  pos_y/1 -> Vector Concatenate/2
  Vector Concatenate/1 -> pos_2d/1
  pos_x/1 -> Vector Concatenate/1
  "sensor_dir (-1,0,1) "/1 -> Compare To Zero/1, "vector rotation "/3(y_dir)
  "theta "/1 -> "vector rotation "/1(angle)
  Compare To Zero/1 -> Switch/2
  Constant/1 -> Switch/1
  Constant1/1 -> Switch/3
  Switch/1 -> "vector rotation "/2(x_dir)

== system model/generate_proximity_sensor_readings/sensor_ray_generation left ==
  "theta " : Inport
  pos_x : Inport  Port=2
  pos_y : Inport  Port=3
  "sensor_dir (-1,0,1) " : Inport  Port=4
  Compare To Zero : simulink/Logic and Bit Operations/Compare To Zero  relop===  OutDataTypeStr=boolean
  Constant : Constant  Value=1.0
  Constant1 : Constant  Value=0
  Switch : Switch  Threshold=1
  Vector Concatenate : Concatenate
  "vector rotation " : Subsystem
  pos_2d : Outport
  "sensor_ray " : Outport  Port=2
  wires:
  Switch/1 -> "vector rotation "/2(x_dir)
  Constant1/1 -> Switch/3
  Constant/1 -> Switch/1
  Compare To Zero/1 -> Switch/2
  "theta "/1 -> "vector rotation "/1(angle)
  "sensor_dir (-1,0,1) "/1 -> "vector rotation "/3(y_dir), Compare To Zero/1
  pos_x/1 -> Vector Concatenate/1
  Vector Concatenate/1 -> pos_2d/1
  pos_y/1 -> Vector Concatenate/2
  "vector rotation "/1("rotated_vector ") -> "sensor_ray "/1

== system model/generate_proximity_sensor_readings/sensor_ray_generation right ==
  "theta " : Inport
  pos_x : Inport  Port=2
  pos_y : Inport  Port=3
  "sensor_dir (-1,0,1) " : Inport  Port=4
  Compare To Zero : simulink/Logic and Bit Operations/Compare To Zero  relop===  OutDataTypeStr=boolean
  Constant : Constant  Value=1.0
  Constant1 : Constant  Value=0
  Switch : Switch  Threshold=1
  Vector Concatenate : Concatenate
  "vector rotation " : Subsystem
  pos_2d : Outport
  "sensor_ray " : Outport  Port=2
  wires:
  "vector rotation "/1("rotated_vector ") -> "sensor_ray "/1
  pos_y/1 -> Vector Concatenate/2
  Vector Concatenate/1 -> pos_2d/1
  pos_x/1 -> Vector Concatenate/1
  "sensor_dir (-1,0,1) "/1 -> Compare To Zero/1, "vector rotation "/3(y_dir)
  "theta "/1 -> "vector rotation "/1(angle)
  Compare To Zero/1 -> Switch/2
  Constant/1 -> Switch/1
  Constant1/1 -> Switch/3
  Switch/1 -> "vector rotation "/2(x_dir)

== system model/Collector A/referee_update_handler1/1 if positive, 2 if negative ==
  In1 : Inport
  Constant1 : Constant  Value=0
  Constant9 : Constant
  Subsystem : Subsystem
  Switch1 : Switch  Criteria=u2 > Threshold
  Out1 : Outport
  wires:
  Constant9/1 -> Switch1/1
  In1/1 -> Switch1/2, Subsystem/1(Input)
  Switch1/1 -> Subsystem/Enable
  Subsystem/1(Output) -> Out1/1
  Constant1/1 -> Switch1/3

== system model/Collector A/referee_update_handler1/Subsystem1 ==
  In1 : Inport
  Constant : Constant  Value=0
  Constant9 : Constant
  Subsystem : Subsystem
  Switch1 : Switch  Criteria=u2 > Threshold
  Out1 : Outport
  wires:
  Constant9/1 -> Switch1/1
  In1/1 -> Switch1/2, Subsystem/1(Input)
  Switch1/1 -> Subsystem/Enable
  Subsystem/1(Output) -> Out1/1
  Constant/1 -> Switch1/3

== system model/Collector A/referee_update_handler1/Subsystem2 ==
  In1 : Inport
  Constant : Constant  Value=0
  Constant9 : Constant
  Subsystem : Subsystem
  Switch1 : Switch  Criteria=u2 > Threshold
  Out1 : Outport
  wires:
  Constant9/1 -> Switch1/1
  In1/1 -> Switch1/2, Subsystem/1(Input)
  Switch1/1 -> Subsystem/Enable
  Subsystem/1(Output) -> Out1/1
  Constant/1 -> Switch1/3

== system model/Collector A/referee_update_handler1/Subsystem3 ==
  In1 : Inport
  Constant : Constant  Value=0
  Constant9 : Constant
  Subsystem : Subsystem
  Switch1 : Switch  Criteria=u2 > Threshold
  Out1 : Outport
  wires:
  Constant9/1 -> Switch1/1
  In1/1 -> Switch1/2, Subsystem/1(Input)
  Switch1/1 -> Subsystem/Enable
  Subsystem/1(Output) -> Out1/1
  Constant/1 -> Switch1/3

== system model/Collector A/referee_update_handler1/Subsystem4 ==
  In1 : Inport
  Constant : Constant  Value=0
  Constant9 : Constant
  Subsystem : Subsystem
  Switch1 : Switch  Criteria=u2 > Threshold
  Out1 : Outport
  wires:
  Constant9/1 -> Switch1/1
  In1/1 -> Switch1/2, Subsystem/1(Input)
  Switch1/1 -> Subsystem/Enable
  Subsystem/1(Output) -> Out1/1
  Constant/1 -> Switch1/3

== system model/Scout A/referee_update_handler/1 if positive, 2 if negative ==
  In1 : Inport
  Constant : Constant  Value=0
  Constant9 : Constant
  Subsystem : Subsystem
  Switch1 : Switch  Criteria=u2 > Threshold
  Out1 : Outport
  wires:
  Constant9/1 -> Switch1/1
  In1/1 -> Switch1/2, Subsystem/1(Input)
  Switch1/1 -> Subsystem/Enable
  Subsystem/1(Output) -> Out1/1
  Constant/1 -> Switch1/3

== system model/Scout A/referee_update_handler/Subsystem1 ==
  In1 : Inport
  Constant : Constant  Value=0
  Constant9 : Constant
  Subsystem : Subsystem
  Switch1 : Switch  Criteria=u2 > Threshold
  Out1 : Outport
  wires:
  Constant9/1 -> Switch1/1
  In1/1 -> Switch1/2, Subsystem/1(Input)
  Switch1/1 -> Subsystem/Enable
  Subsystem/1(Output) -> Out1/1
  Constant/1 -> Switch1/3

== system model/Scout A/referee_update_handler/Subsystem2 ==
  In1 : Inport
  Constant : Constant  Value=0
  Constant9 : Constant
  Subsystem : Subsystem
  Switch1 : Switch  Criteria=u2 > Threshold
  Out1 : Outport
  wires:
  Constant9/1 -> Switch1/1
  In1/1 -> Switch1/2, Subsystem/1(Input)
  Switch1/1 -> Subsystem/Enable
  Subsystem/1(Output) -> Out1/1
  Constant/1 -> Switch1/3

== system model/Scout A/referee_update_handler/Subsystem3 ==
  In1 : Inport
  Constant1 : Constant  Value=0
  Constant9 : Constant
  Subsystem : Subsystem
  Switch1 : Switch  Criteria=u2 > Threshold
  Out1 : Outport
  wires:
  Constant9/1 -> Switch1/1
  In1/1 -> Switch1/2, Subsystem/1(Input)
  Switch1/1 -> Subsystem/Enable
  Subsystem/1(Output) -> Out1/1
  Constant1/1 -> Switch1/3

== system model/Scout A/referee_update_handler/Subsystem4 ==
  In1 : Inport
  Constant1 : Constant  Value=0
  Constant9 : Constant
  Subsystem : Subsystem
  Switch1 : Switch  Criteria=u2 > Threshold
  Out1 : Outport
  wires:
  Constant9/1 -> Switch1/1
  In1/1 -> Switch1/2, Subsystem/1(Input)
  Switch1/1 -> Subsystem/Enable
  Subsystem/1(Output) -> Out1/1
  Constant1/1 -> Switch1/3

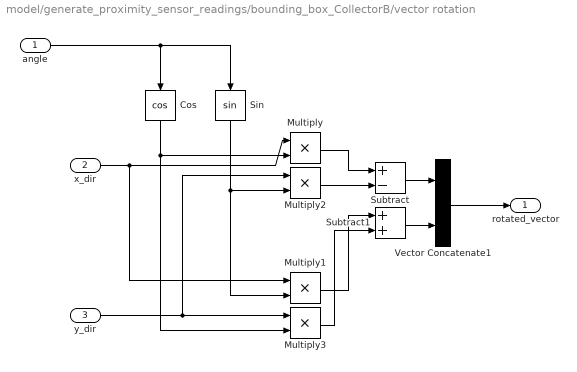
== system model/generate_proximity_sensor_readings/bounding_box_CollectorB/vector rotation  ==
  angle : Inport
  x_dir : Inport  Port=2
  y_dir : Inport  Port=3
  Cos : Trigonometry  Operator=cos
  Multiply{,1..3} (4 alike) : Product
  Sin : Trigonometry
  Subtract : Sum  Inputs=+-
  Subtract1 : Sum
  Vector Concatenate1 : Concatenate
  "rotated_vector " : Outport
  wires:
  Multiply2/1 -> Subtract/2
  Subtract/1 -> Vector Concatenate1/1
  Vector Concatenate1/1 -> "rotated_vector "/1
  x_dir/1 -> Multiply/1, Multiply1/1
  angle/1 -> Sin/1, Cos/1
  Sin/1 -> Multiply2/2, Multiply1/2
  Cos/1 -> Multiply/2, Multiply3/2
  Subtract1/1 -> Vector Concatenate1/2
  y_dir/1 -> Multiply2/1, Multiply3/1
  Multiply/1 -> Subtract/1
  Multiply1/1 -> Subtract1/1
  Multiply3/1 -> Subtract1/2

== system model/generate_proximity_sensor_readings/bounding_box_CollectorB/vector rotation 1 ==
  angle : Inport
  x_dir : Inport  Port=2
  y_dir : Inport  Port=3
  Cos : Trigonometry  Operator=cos
  Multiply{,1..3} (4 alike) : Product
  Sin : Trigonometry
  Subtract : Sum  Inputs=+-
  Subtract1 : Sum
  Vector Concatenate1 : Concatenate
  "rotated_vector " : Outport
  wires:
  Multiply3/1 -> Subtract1/2
  Multiply1/1 -> Subtract1/1
  Multiply/1 -> Subtract/1
  y_dir/1 -> Multiply3/1, Multiply2/1
  Subtract1/1 -> Vector Concatenate1/2
  Cos/1 -> Multiply3/2, Multiply/2
  Sin/1 -> Multiply1/2, Multiply2/2
  angle/1 -> Cos/1, Sin/1
  x_dir/1 -> Multiply1/1, Multiply/1
  Vector Concatenate1/1 -> "rotated_vector "/1
  Subtract/1 -> Vector Concatenate1/1
  Multiply2/1 -> Subtract/2

== system model/generate_proximity_sensor_readings/bounding_box_ScoutA/vector rotation  ==
  angle : Inport
  x_dir : Inport  Port=2
  y_dir : Inport  Port=3
  Cos : Trigonometry  Operator=cos
  Multiply{,1..3} (4 alike) : Product
  Sin : Trigonometry
  Subtract : Sum  Inputs=+-
  Subtract1 : Sum
  Vector Concatenate1 : Concatenate
  "rotated_vector " : Outport
  wires:
  Multiply2/1 -> Subtract/2
  Subtract/1 -> Vector Concatenate1/1
  Vector Concatenate1/1 -> "rotated_vector "/1
  x_dir/1 -> Multiply/1, Multiply1/1
  angle/1 -> Sin/1, Cos/1
  Sin/1 -> Multiply2/2, Multiply1/2
  Cos/1 -> Multiply/2, Multiply3/2
  Subtract1/1 -> Vector Concatenate1/2
  y_dir/1 -> Multiply2/1, Multiply3/1
  Multiply/1 -> Subtract/1
  Multiply1/1 -> Subtract1/1
  Multiply3/1 -> Subtract1/2

== system model/generate_proximity_sensor_readings/bounding_box_ScoutA/vector rotation 1 ==
  angle : Inport
  x_dir : Inport  Port=2
  y_dir : Inport  Port=3
  Cos : Trigonometry  Operator=cos
  Multiply{,1..3} (4 alike) : Product
  Sin : Trigonometry
  Subtract : Sum  Inputs=+-
  Subtract1 : Sum
  Vector Concatenate1 : Concatenate
  "rotated_vector " : Outport
  wires:
  Multiply3/1 -> Subtract1/2
  Multiply1/1 -> Subtract1/1
  Multiply/1 -> Subtract/1
  y_dir/1 -> Multiply3/1, Multiply2/1
  Subtract1/1 -> Vector Concatenate1/2
  Cos/1 -> Multiply3/2, Multiply/2
  Sin/1 -> Multiply1/2, Multiply2/2
  angle/1 -> Cos/1, Sin/1
  x_dir/1 -> Multiply1/1, Multiply/1
  Vector Concatenate1/1 -> "rotated_vector "/1
  Subtract/1 -> Vector Concatenate1/1
  Multiply2/1 -> Subtract/2

== system model/generate_proximity_sensor_readings/bounding_box_ScoutB/vector rotation  ==
  angle : Inport
  x_dir : Inport  Port=2
  y_dir : Inport  Port=3
  Cos : Trigonometry  Operator=cos
  Multiply{,1..3} (4 alike) : Product
  Sin : Trigonometry
  Subtract : Sum  Inputs=+-
  Subtract1 : Sum
  Vector Concatenate1 : Concatenate
  "rotated_vector " : Outport
  wires:
  Multiply3/1 -> Subtract1/2
  Multiply1/1 -> Subtract1/1
  Multiply/1 -> Subtract/1
  y_dir/1 -> Multiply3/1, Multiply2/1
  Subtract1/1 -> Vector Concatenate1/2
  Cos/1 -> Multiply3/2, Multiply/2
  Sin/1 -> Multiply1/2, Multiply2/2
  angle/1 -> Cos/1, Sin/1
  x_dir/1 -> Multiply1/1, Multiply/1
  Vector Concatenate1/1 -> "rotated_vector "/1
  Subtract/1 -> Vector Concatenate1/1
  Multiply2/1 -> Subtract/2

== system model/generate_proximity_sensor_readings/bounding_box_ScoutB/vector rotation 1 ==
  angle : Inport
  x_dir : Inport  Port=2
  y_dir : Inport  Port=3
  Cos : Trigonometry  Operator=cos
  Multiply{,1..3} (4 alike) : Product
  Sin : Trigonometry
  Subtract : Sum  Inputs=+-
  Subtract1 : Sum
  Vector Concatenate1 : Concatenate
  "rotated_vector " : Outport
  wires:
  Multiply2/1 -> Subtract/2
  Subtract/1 -> Vector Concatenate1/1
  Vector Concatenate1/1 -> "rotated_vector "/1
  x_dir/1 -> Multiply/1, Multiply1/1
  angle/1 -> Sin/1, Cos/1
  Sin/1 -> Multiply2/2, Multiply1/2
  Cos/1 -> Multiply/2, Multiply3/2
  Subtract1/1 -> Vector Concatenate1/2
  y_dir/1 -> Multiply2/1, Multiply3/1
  Multiply/1 -> Subtract/1
  Multiply1/1 -> Subtract1/1
  Multiply3/1 -> Subtract1/2

== system model/generate_proximity_sensor_readings/sensor_ray_generation front/vector rotation  ==
  angle : Inport
  x_dir : Inport  Port=2
  y_dir : Inport  Port=3
  Cos : Trigonometry  Operator=cos
  Multiply{,1..3} (4 alike) : Product
  Sin : Trigonometry
  Subtract : Sum  Inputs=+-
  Subtract1 : Sum
  Vector Concatenate1 : Concatenate
  "rotated_vector " : Outport
  wires:
  Multiply3/1 -> Subtract1/2
  Multiply1/1 -> Subtract1/1
  Multiply/1 -> Subtract/1
  y_dir/1 -> Multiply3/1, Multiply2/1
  Subtract1/1 -> Vector Concatenate1/2
  Cos/1 -> Multiply3/2, Multiply/2
  Sin/1 -> Multiply1/2, Multiply2/2
  angle/1 -> Cos/1, Sin/1
  x_dir/1 -> Multiply1/1, Multiply/1
  Vector Concatenate1/1 -> "rotated_vector "/1
  Subtract/1 -> Vector Concatenate1/1
  Multiply2/1 -> Subtract/2

== system model/generate_proximity_sensor_readings/sensor_ray_generation left/vector rotation  ==
  angle : Inport
  x_dir : Inport  Port=2
  y_dir : Inport  Port=3
  Cos : Trigonometry  Operator=cos
  Multiply{,1..3} (4 alike) : Product
  Sin : Trigonometry
  Subtract : Sum  Inputs=+-
  Subtract1 : Sum
  Vector Concatenate1 : Concatenate
  "rotated_vector " : Outport
  wires:
  Multiply2/1 -> Subtract/2
  Subtract/1 -> Vector Concatenate1/1
  Vector Concatenate1/1 -> "rotated_vector "/1
  x_dir/1 -> Multiply/1, Multiply1/1
  angle/1 -> Sin/1, Cos/1
  Sin/1 -> Multiply2/2, Multiply1/2
  Cos/1 -> Multiply/2, Multiply3/2
  Subtract1/1 -> Vector Concatenate1/2
  y_dir/1 -> Multiply2/1, Multiply3/1
  Multiply/1 -> Subtract/1
  Multiply1/1 -> Subtract1/1
  Multiply3/1 -> Subtract1/2

== system model/generate_proximity_sensor_readings/sensor_ray_generation right/vector rotation  ==
  angle : Inport
  x_dir : Inport  Port=2
  y_dir : Inport  Port=3
  Cos : Trigonometry  Operator=cos
  Multiply{,1..3} (4 alike) : Product
  Sin : Trigonometry
  Subtract : Sum  Inputs=+-
  Subtract1 : Sum
  Vector Concatenate1 : Concatenate
  "rotated_vector " : Outport
  wires:
  Multiply3/1 -> Subtract1/2
  Multiply1/1 -> Subtract1/1
  Multiply/1 -> Subtract/1
  y_dir/1 -> Multiply3/1, Multiply2/1
  Subtract1/1 -> Vector Concatenate1/2
  Cos/1 -> Multiply3/2, Multiply/2
  Sin/1 -> Multiply1/2, Multiply2/2
  angle/1 -> Cos/1, Sin/1
  x_dir/1 -> Multiply1/1, Multiply/1
  Vector Concatenate1/1 -> "rotated_vector "/1
  Subtract/1 -> Vector Concatenate1/1
  Multiply2/1 -> Subtract/2

== system model/Collector A/referee_update_handler1/1 if positive, 2 if negative/Subsystem ==
  Input : Inport
  Enable : EnablePort
  Output : Outport
  wires:
  Input/1 -> Output/1

== system model/Collector A/referee_update_handler1/Subsystem1/Subsystem ==
  Input : Inport
  Enable : EnablePort
  Output : Outport
  wires:
  Input/1 -> Output/1

== system model/Collector A/referee_update_handler1/Subsystem2/Subsystem ==
  Input : Inport
  Enable : EnablePort
  Output : Outport
  wires:
  Input/1 -> Output/1

== system model/Collector A/referee_update_handler1/Subsystem3/Subsystem ==
  Input : Inport
  Enable : EnablePort
  Output : Outport
  wires:
  Input/1 -> Output/1

== system model/Collector A/referee_update_handler1/Subsystem4/Subsystem ==
  Input : Inport
  Enable : EnablePort
  Output : Outport
  wires:
  Input/1 -> Output/1

== system model/Scout A/referee_update_handler/1 if positive, 2 if negative/Subsystem ==
  Input : Inport
  Enable : EnablePort
  Output : Outport
  wires:
  Input/1 -> Output/1

== system model/Scout A/referee_update_handler/Subsystem1/Subsystem ==
  Input : Inport
  Enable : EnablePort
  Output : Outport
  wires:
  Input/1 -> Output/1

== system model/Scout A/referee_update_handler/Subsystem2/Subsystem ==
  Input : Inport
  Enable : EnablePort
  Output : Outport
  wires:
  Input/1 -> Output/1

== system model/Scout A/referee_update_handler/Subsystem3/Subsystem ==
  Input : Inport
  Enable : EnablePort
  Output : Outport
  wires:
  Input/1 -> Output/1

== system model/Scout A/referee_update_handler/Subsystem4/Subsystem ==
  Input : Inport
  Enable : EnablePort
  Output : Outport
  wires:
  Input/1 -> Output/1
